simulink model "Experiment_2"  (R2017b)
settings: Solver=ode4  StartTime=0.0  StopTime=inf  FixedStep=0.0001  RelTol=1e-3
PostLoadFcn:
  | , if any(exist('dsrtsu_mdlpostloadfcn', 'file') == [2, 3, 6]), try dsrtsu_mdlpostloadfcn('Execute', bdroot); catch fprintf('Error in PostLoadFcn (dsrtsu_mdlpostloadfcn) for model "%s":\n %s\n', bdroot, lasterr); end, end,
libraries: rtilib1104 x3, dspstat3 x1
settings Model: DSRTSU_INTERNAL_RTI_VER=510  DSRTSU_INTERNAL_RTI_TYPE=rti1104  RTICANMMDATA=struct('GeneralSetupData',struct('modelroot','\\depot.engr.oregonstate.edu\users\garciafv\Windows.Documents\Desktop\ECE_332\Lab2','generalsettings',struct('filesettings',struct('destfolder',struct('Name','RTICANMM_FILES','Check',1),'buildfolder',struct('Name','.','Check',1),'AbsDestfolder',struct('Name','\\depot.engr.oregonstate.edu\users\garciafv\Windows.Documents\Desktop\ECE_332\Lab2\RTICANMM_FILES'),'AbsBuildfolder',struct('Name','\\depot.engr.oregonstate.edu\users\garciafv\Windows.Documents\Desktop\ECE_332\Lab2'))),'options',struct('addpaths',1,'rmpaths',1,'addtrcexclusion',logical(1),'cannavigator',struct('checkmonitoring',0),'show_usrtrc',0,'use_usrtrc',0),'advanced',struct('options',[1 1 1 1 1 1 1 1 1 1 1 1 1 1 1 1 1 1 1 1 1 1 1 1 1 1 1 1 1 1 1 1 1 1 1 1 1 1 1 1 1 1 1 1 1 1 1 1 1 1 1 1 1 1 1 1 1 1 1 1 1 1 1 1 1 1 1 1 1 1 1 1 1 1 1 1 1 1 1 1 1 1 1 1 1 1 1 1 1 1 1 1 1 1 1 1 1 1 1 1]),'MPSetup',{{}},'modelname','Experiment_2','block','Experiment_2'))  DSRTSU_INTERNAL_RTIFLEXRAYCONFIG=110  DSRTSU_INTERNAL_RTIFPGA=110  Creator=garciafv  LastModifiedBy=garciafv
settings OptimizationCC: BlockReduction=off
settings HardwareCC: ProdBitPerPointer=32  ProdBitPerSizeT=32  ProdBitPerPtrDiffT=32  ProdLargestAtomicInteger=Integer  ProdEndianess=BigEndian  ProdWordSize=32  ProdHWDeviceType=Custom Processor->Custom  TargetIntDivRoundTo=Zero  TargetEndianess=BigEndian  TargetHWDeviceType=Custom Processor->Custom
settings SFSimCC: MATLABDynamicMemAlloc=off
settings RTWCC: SystemTargetFile=rti1104.tlc  MakeCommand=make_rti  TemplateMakefile=rti1104.tmf  Description=dSPACE DS1104 Hardware Platform
settings STFCustomTargetCC: ParMdlRefBuildCompliant=on  GRTInterface=off  SystemTargetFile=rti1104.tlc
settings GRTTargetCC: TargetLangStandard=C89/C90 (ANSI)  CompOptLevelCompliant=off  ConcurrentExecutionCompliant=off  CombineOutputUpdateFcns=off  MatFileLogging=off  CPPClassGenCompliant=off  UseToolchainInfoCompliant=off

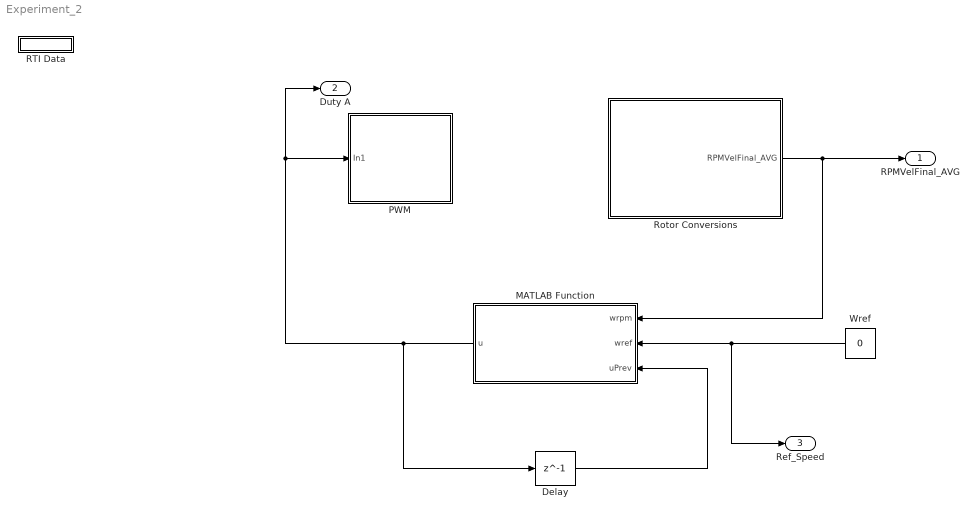
== system Experiment_2 ==
  Delay : Delay  DelayLength=1
  MATLAB Function : MATLAB Function  TreatAsAtomicUnit=on
  PWM : Subsystem
  RTI Data : Subsystem  Tag=struct('RTIDataServer',struct('RTIDataServerVs','2','RTIModelDescription','struct(''main'',''Experiment_2'',''sub'','''',''isMp'',0)'))  LoadFcn="if exist('rtidc'), try,  rtidc('DataHostBlockClbLoad', gcbh); catch, disp(['Warning: ''LoadFcn'' for RTI Data block failed: ' lasterr]); end, end,"  mask(RTI_DATA_HOST){}
      mask help:
      | RTI Data Block.
      | This block is used by RTI to store internal model-dependent data.
      | Please keep this block on the root level of the model. Deleting this block will result in data loss.
      |
      | NEVER DELETE OR COPY THIS BLOCK!
      settings: CopyFcn="if exist('rtidc'), try,  rtidc('DataHostBlockClbCopy', gcbh); catch, disp(['Warning: ''CopyFcn'' for RTI Data block failed: ' lasterr]); end, end,"  DeleteFcn="if exist('rtidc'), try,  rtidc('DataHostBlockClbDelete', gcbh); catch, disp(['Warning: ''DeleteFcn'' for RTI Data block failed: ' lasterr]); end, end,"  ModelCloseFcn="if exist('rtidc'), try,  rtidc('DataHostBlockClbModelClose', gcbh); catch, disp(['Warning: ''ModelCloseFcn'' for RTI Data block failed: ' lasterr]); end, end,"  PreSaveFcn="if exist('rtidc'), try,  rtidc('DataHostBlockClbPreSave', gcbh); catch, disp(['Warning: ''PreSaveFcn'' for RTI Data block failed: ' lasterr]); end, end,"  PostSaveFcn="if exist('rtidc'), try,  rtidc('DataHostBlockClbPostSave', gcbh); catch, disp(['Warning: ''PostSaveFcn'' for RTI Data block failed: ' lasterr]); end, end,"  NameChangeFcn="if exist('rtidc'), try,  rtidc('DataHostBlockClbNameChange', gcbh); catch, disp(['Warning: ''NameChangeFcn'' for RTI Data block failed: ' lasterr]); end, end,"
      mask Help:
      | RTI Data Block.
      | This block is used by RTI to store internal model-dependent data.
      | Please keep this block on the root level of the model. Deleting this block will result in data loss.
      | 
      | NEVER DELETE OR COPY THIS BLOCK!
      mask Display:
      | text(0.5, 0.5, 'RTI Data', 'HorizontalAlignment', 'center');
      | plot([1 0]);
  Rotor Conversions : Subsystem
  Wref : Constant  Value=0
  RPMVelFinal_AVG : Outport
  Duty A : Outport  Port=2
  Ref_Speed : Outport  Port=3
  wires:
  Rotor Conversions/1(RPMVelFinal_AVG) -> MATLAB Function/1(wrpm), RPMVelFinal_AVG/1
  MATLAB Function/1(u) -> Delay/1, Duty A/1, PWM/1(In1)
  Wref/1 -> MATLAB Function/2(wref), Ref_Speed/1
  Delay/1 -> MATLAB Function/3(uPrev)

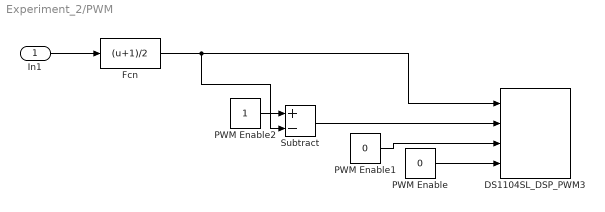
== system Experiment_2/PWM ==
  In1 : Inport
  DS1104SL_DSP_PWM3 : rtilib1104/DS1104 SLAVE DSP/DS1104SL_DSP_PWM3  Parameters=[]  TDef=[]  BoardType=[]  PwmMode=[]  Frequency=[]  DeadBand=[]  InitValue=[]  TermMode=[]  TermValue=[]  IntDelay=[]  DialogFcn=[]  Reserved1=[]  Reserved2=[]  Reserved3=[]  Reserved4=[]  Revision=[]  UnitName=[]  UnitValues=[]  DSProperties=struct('RTI',struct('Version',uint32(2),'BlockType',struct('isSLSource',uint8(0),'isSLSink',uint8(1),'isHWSource',uint8(0),'isHWSink',uint8(1),'isSetup',uint8(0),'isInline',uint8(1),'isNonInline',uint8(0),'isInterrupt',uint8(0),'isChannelwise',uint8(0)),'IOBoardType','DS1104SLAVE','UnitType','PWM','Identifier','PWM3','DialogType','ML','BlockSet','NONE','SlaveProcessor','F240'))  RTIBlockInterface=struct('InputPortsActive',[1 1 1 1],'InputPortsWidth',int32([1 1 1 1]),'InputPortsName',{{['Duty cycle a'],['Duty cycle b'],['Duty cycle c'],['PWM Stop']}},'IWork',{{{'',uint32(1)}}},'DialogFcn','rti1104slavepwm3gui','InitLevel',1,'BlockDisplay',{{'','auto'}},'IconTransparency','on','BlockName',struct('Token',{{'DS1104SL_DSP_PWM3'}}))  RTIBlockParameters=struct('PWMFrequency',{{'20000','OFF',[]}},'PWMDeadband',{{'1','OFF',[]}},'PWMPolarityMode',{{[1 1 1 1],'OFF',[]}},'PWMPolarityInvMode',{{[2 2 2 2],'OFF',[]}},'SuspendModeInit',{{[1 1 1],'OFF',[]}},'TTLModeInit',{{[2 2 2],'OFF',[]}},'TTLModeInitNOT',{{[1 1 1],'OFF',[]}},'DutyCycleInitValueCh1',{{'0.5','OFF',[]}},'DutyCycleInitValueCh2',{{'0.5','OFF',[]}},'DutyCycleInitValueCh3',{{'0.5','OFF',[]}},'EnablePWMStop',{{1,'OFF',[]}},'SuspendModeTerm',{{[1 1 1],'OFF',[]}},'TTLModeTerm',{{[2 2 2],'OFF',[]}},'TTLModeTermNOT',{{[1 1 1],'OFF',[]}},'DutyCycleTermValueCh1',{{'0.5','OFF',[]}},'DutyCycleTermValueCh2',{{'0.5','OFF',[]}},'DutyCycleTermValueCh3',{{'0.5','OFF',[]}},'TLCFileName',{{'rti1104pwm3','OFF',[]}})  RTISFcnParameters=struct('PWMFrequency','double','PWMDeadband','double','PWMPolarityMode','double','PWMPolarityInvMode','double','SuspendModeInit','double','TTLModeInit','double','TTLModeInitNOT','double','DutyCycleInitValueCh1','double','DutyCycleInitValueCh2','double','DutyCycleInitValueCh3','double','EnablePWMStop','double','SuspendModeTerm','double','TTLModeTerm','double','TTLModeTermNOT','double','DutyCycleTermValueCh1','double','DutyCycleTermValueCh2','double','DutyCycleTermValueCh3','double','TLCFileName','char')  RTIBlockParaDefault=struct('PWMFrequency',100,'PWMDeadband',50,'PWMPolarityMode',[1 1 1 1],'PWMPolarityInvMode',[2 2 2 2],'SuspendModeInit',[1 1 1],'TTLModeInit',[2 2 2],'TTLModeInitNOT',[1 1 1],'DutyCycleInitValueCh1',2^-1,'DutyCycleInitValueCh2',2^-1,'DutyCycleInitValueCh3',2^-1,'EnablePWMStop',1,'SuspendModeTerm',[1 1 1],'TTLModeTerm',[2 2 2],'TTLModeTermNOT',[1 1 1],'DutyCycleTermValueCh1',2^-1,'DutyCycleTermValueCh2',2^-1,'DutyCycleTermValueCh3',2^-1,'TLCFileName','rti1104pwm3')
      settings: SourceProductName=dSPACE RTI1104
  Fcn : Fcn  Expr=(u+1)/2
  PWM Enable : Constant  Value=0
  PWM Enable1 : Constant  Value=0
  PWM Enable2 : Constant
  Subtract : Sum  Inputs=+-
  wires:
  In1/1 -> Fcn/1
  Subtract/1 -> DS1104SL_DSP_PWM3/2
  PWM Enable/1 -> DS1104SL_DSP_PWM3/4
  PWM Enable1/1 -> DS1104SL_DSP_PWM3/3
  Fcn/1 -> Subtract/2, DS1104SL_DSP_PWM3/1
  PWM Enable2/1 -> Subtract/1

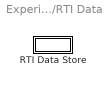
== system Experiment_2/RTI Data ==
  RTI Data Store : Subsystem  Tag="struct('private',struct('version',struct('dsVer',uint32(2),'dsVerCreation',uint32(2),'RTI',struct('ver','7.9','type','RTI1104')),'access',struct('type','Model','isPerm',1,'created',['24-Jan-2020 12:31:47'],'modified',['13-Mar-2020 12:02:47'],'location','')),'public',struct('main',struct('data',[]),'sub',struct('name',{{'Experiment_2'}},'data',{{struct('TH',struct('thTaskInfo',struct('taskType',{'TIMER','HWINT','TMRINT','SWINT','GLINT'},'tasksNumOf',{1,0,0,0,0},'srcIds',{{'TIMERA'},{},{},{},{}},'taskNames',{{['Timer Task 1']},{},{},{},{}})),'th_tc',struct('dataType','TASK','taskGroupId','','taskGroupList',{{}},'taskSchedulingPolicy','FCFS','taskType','TIMER','blkh',-1,'srcId','TIMERA','srcSgnName',['Timer A interrupt'],'srcCpuName','','taskName',['Timer Task 1  [0.0001] s'],'taskNameDisplayExt','','smplTime',0.0001,'smplTimeOffs',0,'hasFixedPriority',0,'priority',1,'hasFixedOvc',0,'ovcType',1,'ovcMax',1),'tc_th',struct('dataType','TASK','taskGroupId','','taskGroupList',{{}},'taskSchedulingPolicy','FCFS','taskType','TIMER','blkh',-1,'srcId','TIMERA','srcSgnName',['Timer A interrupt'],'srcCpuName','','taskName',['Timer Task 1  [0.0001] s'],'taskNameDisplayExt','','smplTime',0.0001,'smplTimeOffs',0,'hasFixedPriority',0,'priority',1,'hasFixedOvc',0,'ovcType',1,'ovcMax',1))}})))"  mask(RTI_DATA_STORE){}
      mask help:
      | RTI Data Store Block. This block is used by RTI to store internal model dependent data. Deleting this block will result in data loss.
      |
      | NEVER DELETE, COPY, OR MODIFY THIS BLOCK!
      mask Help:
      | RTI Data Store Block. This block is used by RTI to store internal model dependent data. Deleting this block will result in data loss.
      | 
      | NEVER DELETE, COPY, OR MODIFY THIS BLOCK!
      mask Display: text(0.5, 0.5, ' ', 'HorizontalAlignment', 'center');

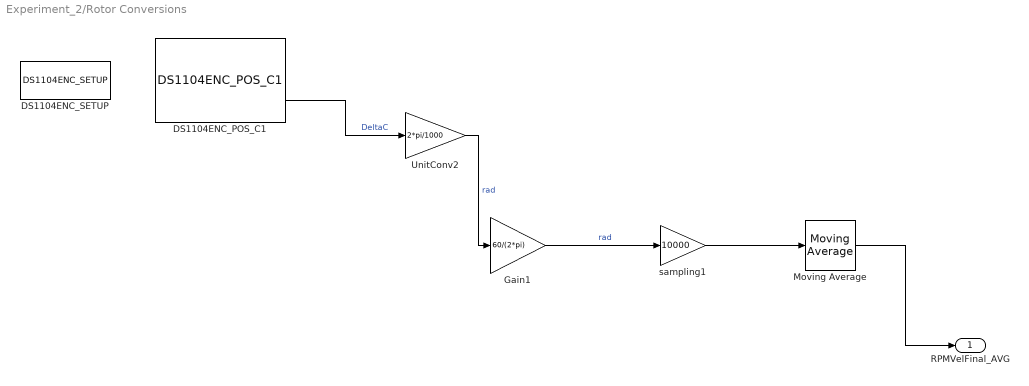
== system Experiment_2/Rotor Conversions ==
  DS1104ENC_POS_C1 : rtilib1104/DS1104 MASTER PPC/DS1104ENC_POS_C1  ChannelNo=1  PosValue=0  Reserved1=[]  Reserved2=[]  Reserved3=[]  Reserved4=[]  DialogFcn=gui1104enc_pos  UnitName={'DS1104ENC_POS_C'}  UnitValues={ 1 }  DSProperties=struct('RTI',struct('Version',uint32(1),'BlockType',struct('isSLSource',uint8(1),'isSLSink',uint8(0),'isHWSource',uint8(1),'isHWSink',uint8(0),'isSetup',uint8(0),'isInline',uint8(1),'isNonInline',uint8(0),'isInterrupt',uint8(0),'isChannelwise',uint8(1)),'IOBoardType','DS1104MASTER','UnitType','ENC','Identifier','ENCPOSCH','DialogType','ML','BlockSet','NONE','SlaveProcessor','NONE'))
      settings: SourceProductName=dSPACE RTI1104
  DS1104ENC_SETUP : rtilib1104/DS1104 MASTER PPC/DS1104ENC_SETUP  Reserved1=[]  Reserved2=[]  Reserved3=[]  Reserved4=[]  DialogFcn=gui1104enc_setup  UnitName={'DS1104ENC_SETUP'}  UnitValues={ [] }  DSProperties=struct('RTI',struct('Version',uint32(1),'BlockType',struct('isSLSource',uint8(0),'isSLSink',uint8(0),'isHWSource',uint8(0),'isHWSink',uint8(0),'isSetup',uint8(0),'isInline',uint8(1),'isNonInline',uint8(0),'isInterrupt',uint8(0),'isChannelwise',uint8(0)),'IOBoardType','DS1104MASTER','UnitType','ENC','Identifier','ENCSETUP','DialogType','ML','BlockSet','NONE','SlaveProcessor','NONE'))
      settings: SourceProductName=dSPACE RTI1104  SignalType=[0 0]
  Gain1 : Gain  Gain=60/(2*pi)
  Moving Average : dspstat3/Moving Average  Method=Sliding window  SpecifyWindowLength=on  WindowLength=25  ForgettingFactor=0.9  SimulateUsing=Code generation
  UnitConv2 : Gain  Gain=2*pi/1000
  sampling1 : Gain  Gain=10000
  RPMVelFinal_AVG : Outport
  wires:
  Gain1/1 -> sampling1/1  "rad"
  sampling1/1 -> Moving Average/1
  Moving Average/1 -> RPMVelFinal_AVG/1
  UnitConv2/1 -> Gain1/1  "rad"
  DS1104ENC_POS_C1/2 -> UnitConv2/1  "DeltaC"

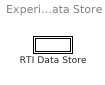
== system Experiment_2/RTI Data/RTI Data Store ==
  RTI Data Store : Subsystem  mask(RTI_DATA_STORE){}
      mask help:
      | RTI Data Store Block. This block is used by RTI to store internal model dependent data. Deleting this block will result in data loss.
      |
      | NEVER DELETE, COPY, OR MODIFY THIS BLOCK!
      mask Help:
      | RTI Data Store Block. This block is used by RTI to store internal model dependent data. Deleting this block will result in data loss.
      | 
      | NEVER DELETE, COPY, OR MODIFY THIS BLOCK!
      mask Display: text(0.5, 0.5, ' ', 'HorizontalAlignment', 'center');

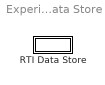
== system Experiment_2/RTI Data/RTI Data Store/RTI Data Store ==
  RTI Data Store : Subsystem  mask(RTI_DATA_STORE){}
      mask help:
      | RTI Data Store Block. This block is used by RTI to store internal model dependent data. Deleting this block will result in data loss.
      |
      | NEVER DELETE, COPY, OR MODIFY THIS BLOCK!
      mask Help:
      | RTI Data Store Block. This block is used by RTI to store internal model dependent data. Deleting this block will result in data loss.
      | 
      | NEVER DELETE, COPY, OR MODIFY THIS BLOCK!
      mask Display: text(0.5, 0.5, ' ', 'HorizontalAlignment', 'center');

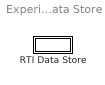
== system Experiment_2/RTI Data/RTI Data Store/RTI Data Store/RTI Data Store ==
  RTI Data Store : Subsystem  mask(RTI_DATA_STORE){}
      mask help:
      | RTI Data Store Block. This block is used by RTI to store internal model dependent data. Deleting this block will result in data loss.
      |
      | NEVER DELETE, COPY, OR MODIFY THIS BLOCK!
      mask Help:
      | RTI Data Store Block. This block is used by RTI to store internal model dependent data. Deleting this block will result in data loss.
      | 
      | NEVER DELETE, COPY, OR MODIFY THIS BLOCK!
      mask Display: text(0.5, 0.5, ' ', 'HorizontalAlignment', 'center');

== system Experiment_2/RTI Data/RTI Data Store/RTI Data Store/RTI Data Store/RTI Data Store ==

== matlab function Experiment_2/MATLAB Function ==
  data: wrpm input; u output; wref input; uPrev input
function u = control(wrpm, wref,uPrev)
    err = wref-wrpm;
    du = .0001
    if err > 0
     u = uPrev+du;
    elseif err < 0
     u = uPrev-du;
    else
      u = uPrev;
    end
    
    if u > 1
        u = 1;
    elseif u < -1
        u = -1;
    end
end
